simulink model "SystemID"  (R2020b)
settings: Solver=ode14x  StartTime=0.0  StopTime=0.4  FixedStep=1e-5  RelTol=1e-6
libraries: fl_lib x4, nesl_utility x4, ee_lib x2
settings Model: Creator=Rodrigo San Roman  LastModifiedBy=DavidZuren

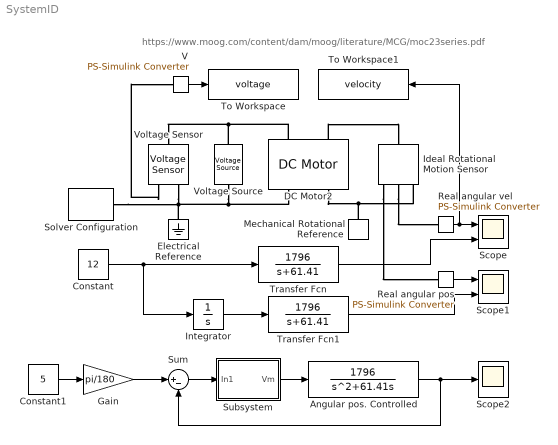
== system SystemID ==
  note: https://www.moog.com/content/dam/moog/literature/MCG/moc23series.pdf
  Angular pos. Controlled : TransferFcn  Numerator=[1796]  Denominator=[1 61.41 0]
  Constant : Constant  Value=12
  Constant1 : Constant  Value=5
  DC Motor2 : ee_lib/Electromechanical/Brushed Motors/DC Motor  field_option=ee.enum.field_option.pm  Rf=100 Ohm  Lf=1 H  Laf=0.15 H  If0=0 A  parameterization=ee.enum.dcparam_option.circuit_param  Ra=0.7 Ohm  La=0.5 mH  emf_or_torque=ee.enum.emf_or_torque.kv  Kv=0.0342 V/(rad/s)  Ki=242 N*m/A  T_stall=0.24e-3 N*m  w_max=19100 rpm  w_rated=15000 rpm  P_rated=0.08 W  V_rated=1.5 V  J=282.5 g*cm^2  lam_param=ee.enum.lam_param.damping  lam=0 N*m/(rad/s)  i_noload=0 A  V_i_noload=1.5 V  speed0=0 rpm  enable_fault_armature=ee.enum.faults.faultEnable.no  rev_faulted=1 / 3  G_faulted_armature=1e-5 S  fault_trigger_armature=ee.enum.faults.faultTrigger.temporal  t_fault_armature=1 s  max_permissible_current_armature=inf A  t_fail_on_current_armature=1 s  enable_fault_field=ee.enum.faults.faultEnable.no  G_faulted_field=1e-5 S  fault_trigger_field=ee.enum.faults.faultTrigger.temporal  t_fault_field=1 s  max_permissible_current_field=inf A  t_fail_on_current_field=1 s  fault_action=ee.enum.faults.faultAction.none  alpha=3.93e-3 1/K  Tmeas=25 degC  thermal_mass=100 J/K  initial_temperature=25 degC
  Electrical Reference : fl_lib/Electrical/Electrical Elements/Electrical Reference
  Gain : Gain  Gain=pi/180
  Ideal Rotational Motion Sensor : fl_lib/Mechanical/Mechanical Sensors/Ideal Rotational Motion Sensor  wrap_angle=simscape.enum.onoff.off  offset=0 rad
  Integrator : Integrator
  Mechanical Rotational Reference : fl_lib/Mechanical/Rotational Elements/Mechanical Rotational Reference
  Real angular pos : nesl_utility/PS-Simulink Converter  PhysicalDomain=network_engine_domain  SubClassName=ps_output  LeftPortType=input  RightPortType=output  PseudoPeriodic=off  Frequencies=[]  Unit=inherit  AffineConversion=off
  Real angular vel : nesl_utility/PS-Simulink Converter  PhysicalDomain=network_engine_domain  SubClassName=ps_output  LeftPortType=input  RightPortType=output  PseudoPeriodic=off  Frequencies=[]  Unit=inherit  AffineConversion=off
  Scope : Scope  NumInputPorts=2
  Scope1 : Scope  NumInputPorts=2
  Scope2 : Scope
  Solver Configuration : nesl_utility/Solver Configuration  PhysicalDomain=network_engine_domain  SubClassName=solver  LeftPortType=input  RightPortType=generic  Tones=[]  Harmonics=[]  SimulateNoise=off  Profile=off  UseLocalSampling=off  EnableSwitchedLinearOptims=on  FrequencyDomain=off  UseCCode=off  RelTol=0.001  AbsTol=1e-06  MinStep=1e-09  ToWorkspace=off  RevertToSquareIcSolve=off  NumHomotopyIterations=100  PhasorMode=off  PhasorModeNumHarmonics=1  DoDC=off  ResidualTolerance=1e-09  UseLocalSolver=off  LocalSolverChoice=NE_BACKWARD_EULER_ADVANCER  LocalSolverSampleTime=0.001  DoFixedCost=off  MaxNonlinIter=3  MaxModeIter=2  ComputeImpulses=off  ImpulseIterations=2  LinearAlgebra=auto  EquationFormulation=NE_TIME_EF  DelaysMemoryBudget=1024  AutomaticFiltering=on  FilteringTimeConstant=0.001  PartitionStorageMethod=AS_NEEDED  PartitionMemoryBudget=1024  PartitionMethod=ROBUST
  Subsystem : Subsystem
  Sum : Sum  Inputs=|+-
  To Workspace : ToWorkspace  VariableName=voltage  SampleTime=-1
  To Workspace1 : ToWorkspace  VariableName=velocity  SampleTime=-1
  Transfer Fcn : TransferFcn  Numerator=[1796]  Denominator=[1 61.41]
  Transfer Fcn1 : TransferFcn  Numerator=[1796]  Denominator=[1 61.41]
  V : nesl_utility/PS-Simulink Converter  PhysicalDomain=network_engine_domain  SubClassName=ps_output  LeftPortType=input  RightPortType=output  PseudoPeriodic=off  Frequencies=[]  Unit=inherit  AffineConversion=off
  Voltage Sensor : fl_lib/Electrical/Electrical Sensors/Voltage Sensor
  Voltage Source : ee_lib/Sources/Voltage Source  dc_voltage=12 V  ac_voltage=0 V  ac_shift=0 rad  ac_frequency=60 Hz  noise_mode=0  PSD=0 V^2/Hz  repeatability=1  auto_seed=3499211588  user_seed=0  sample_time=1e-3 s  i_specify=off  i_priority=None  i=0 A  i_nominal_specify=off  i_nominal_unit=A  i_nominal_value=1  v_specify=off  v_priority=None  v=0 V  v_nominal_specify=off  v_nominal_unit=V  v_nominal_value=1
  wires:
  Real angular vel/1 -> To Workspace1/1, Scope/1
  V/1 -> To Workspace/1
  Constant/1 -> Integrator/1, Transfer Fcn/1
  Transfer Fcn/1 -> Scope/2
  Real angular pos/1 -> Scope1/1
  Integrator/1 -> Transfer Fcn1/1
  Transfer Fcn1/1 -> Scope1/2
  Subsystem/1(Vm) -> Angular pos. Controlled/1
  Angular pos. Controlled/1 -> Sum/2, Scope2/1
  Sum/1 -> Subsystem/1(In1)
  Constant1/1 -> Gain/1
  Gain/1 -> Sum/1
  connections:
  Voltage Source/LConn1 -- Voltage Sensor/LConn1 -- DC Motor2/LConn1
  Voltage Source/RConn1 -- Solver Configuration/RConn1 -- Electrical Reference/LConn1 -- Voltage Sensor/RConn2 -- DC Motor2/RConn1
  Voltage Sensor/RConn1 -- V/LConn1
  DC Motor2/LConn2 -- Ideal Rotational Motion Sensor/LConn1
  DC Motor2/RConn2 -- Mechanical Rotational Reference/LConn1 -- Ideal Rotational Motion Sensor/RConn1
  Ideal Rotational Motion Sensor/RConn2 -- Real angular vel/LConn1
  Ideal Rotational Motion Sensor/RConn3 -- Real angular pos/LConn1

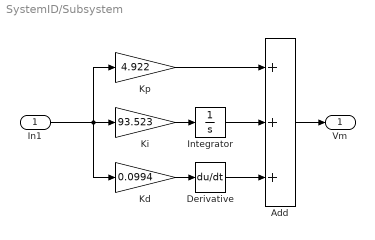
== system SystemID/Subsystem ==
  In1 : Inport
  Add : Sum  Inputs=+++
  Derivative : Derivative
  Integrator : Integrator
  Kd : Gain  Gain=0.0994
  Ki : Gain  Gain=93.523
  Kp : Gain  Gain=4.922
  Vm : Outport
  wires:
  Ki/1 -> Integrator/1
  Add/1 -> Vm/1
  Kp/1 -> Add/1
  Kd/1 -> Derivative/1
  Integrator/1 -> Add/2
  Derivative/1 -> Add/3
  In1/1 -> Ki/1, Kd/1, Kp/1
